simulink model "lab4_model1"  (R2022a)
settings: Solver=VariableStepAuto  StartTime=0.0  StopTime=10.0  RelTol=1e-3
libraries: simulink x4
settings Model: Creator=User  LastModifiedBy=User

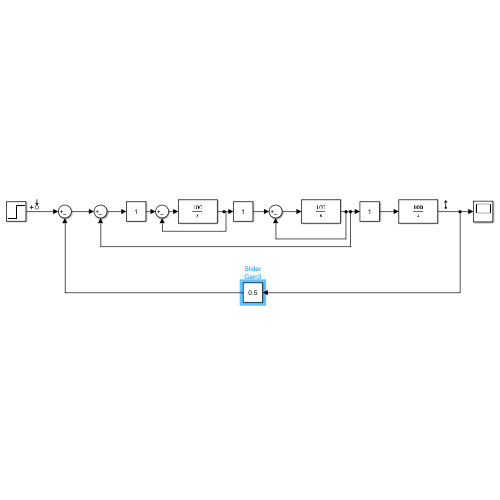
[thumbnail: Simulink's stored preview of the top-level diagram]
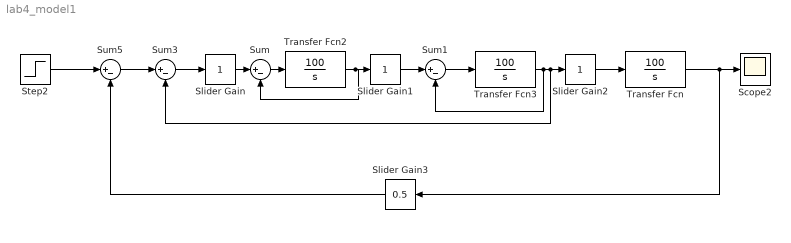
== system lab4_model1 ==
  Scope2 : Scope
  Slider Gain : simulink/Math Operations/Slider Gain  gain=1  low=0  high=2
  Slider Gain1 : simulink/Math Operations/Slider Gain  gain=1  low=0  high=2
  Slider Gain2 : simulink/Math Operations/Slider Gain  gain=1  low=0  high=5
  Slider Gain3 : simulink/Math Operations/Slider Gain  gain=0.5  low=0  high=2
  Step2 : Step  SampleTime=0
  Sum{,1,3,5} (4 alike) : Sum  Inputs=|+-
  Transfer Fcn : TransferFcn  Numerator=[100]  Denominator=[1 0]
  Transfer Fcn2 : TransferFcn  Numerator=[100]  Denominator=[1 0]
  Transfer Fcn3 : TransferFcn  Numerator=[100]  Denominator=[1 0]
  wires:
  Slider Gain/1 -> Sum/1
  Transfer Fcn2/1 -> Sum/2, Slider Gain1/1
  Sum3/1 -> Slider Gain/1
  Sum5/1 -> Sum3/1
  Slider Gain1/1 -> Sum1/1
  Step2/1 -> Sum5/1
  Sum/1 -> Transfer Fcn2/1
  Sum1/1 -> Transfer Fcn3/1
  Transfer Fcn3/1 -> Sum1/2, Sum3/2, Slider Gain2/1
  Slider Gain2/1 -> Transfer Fcn/1
  Transfer Fcn/1 -> Slider Gain3/1, Scope2/1
  Slider Gain3/1 -> Sum5/2
